simulink model "CNcs7"  (Simulink 6.2)
settings: Solver=ode4  SolverMode=SingleTasking  StartTime=0.0  StopTime=5  FixedStep=0.001  MaxStep=0.001  RelTol=1e-3  AbsTol=1e-3
undefined symbols (not defined in the file): alexlaw, bs_onoff, bs_scale, bsfsacrit, bsfsvcrit, cnsgain, fs_onoff, fs_scale, fsdelaycalc, ltdrk, phasicgain, pmcgain, pmctau2, pmctau3, saccrefract, saccsw, spgain, tonicgain, tvrD, tvrN, velnoise, velreconsw
libraries: simulink_extras x38, simulink x2
(part 5 of 5)

== system CNcs7/CN/LMLN  03/03/01/IM CN-LMLN/Saccade Enable/Enable Control/2 ms/leading edge detect ==
  note: leading edge detection
  in_1 : Inport  Port=1  LatchInput=off
  Abs : Abs  SaturateOnIntegerOverflow=on
  Derivative : Derivative
  Relational Operator : RelationalOperator  Operator===  InputSameDT=on
  Sign : Signum
  Threshold 1 : Constant
  out_1 : Outport
  wires:
  Abs/1 -> Derivative/1
  Derivative/1 -> Sign/1
  Sign/1 -> Relational Operator/1
  Threshold 1/1 -> Relational Operator/2
  Relational Operator/1 -> out_1/1
  in_1/1 -> Abs/1

== system CNcs7/CN/LMLN  03/03/01/IM CN-LMLN/Saccade Enable/Enable Control/2 ms/trailing edge detect ==
  note: trailing edge detection
  note: It is also possible to remove the SIGNUM function
      | and the '==', and replace them with a simple
      | switch with a threshold of (say) 150 or so.
  in_1 : Inport  Port=1  LatchInput=off
  Abs : Abs  SaturateOnIntegerOverflow=on
  Derivative : Derivative
  Relational Operator : RelationalOperator  Operator===  InputSameDT=on
  Sign : Signum
  Threshold 1 : Constant  Value=-1
  out_1 : Outport
  wires:
  in_1/1 -> Abs/1
  Relational Operator/1 -> out_1/1
  Threshold 1/1 -> Relational Operator/2
  Sign/1 -> Relational Operator/1
  Derivative/1 -> Sign/1
  Abs/1 -> Derivative/1

== system CNcs7/CN/LMLN  03/03/01/IM CN-LMLN/Saccade Enable/Enable Control/50 ms/SampHold?2 ==
  note: When "S/H?" is LOW, then "Input" is switched directly to the
      | output ("sample").  When "S/H?" is HIGH, the current output is
      | maintained ("hold").
  Input : Inport  Port=1  LatchInput=off
  S/H? : Inport  Port=2  LatchInput=off
  Memory : Memory  Orientation=left
  Sign : Signum
  Switch2 : Switch  Threshold=0.5  SaturateOnIntegerOverflow=on  InputSameDT=on
  output : Outport
  wires:
  S/H?/1 -> Sign/1
  Sign/1 -> Switch2/2
  Input/1 -> Switch2/3
  Switch2/1 -> Memory/1, output/1
  Memory/1 -> Switch2/1

== system CNcs7/CN/LMLN  03/03/01/IM CN-LMLN/Saccade Enable/Enable Control/50 ms/leading edge detect ==
  note: leading edge detection
  in_1 : Inport  Port=1  LatchInput=off
  Abs : Abs  SaturateOnIntegerOverflow=on
  Derivative : Derivative
  Relational Operator : RelationalOperator  Operator===  InputSameDT=on
  Sign : Signum
  Threshold 1 : Constant
  out_1 : Outport
  wires:
  in_1/1 -> Abs/1
  Relational Operator/1 -> out_1/1
  Threshold 1/1 -> Relational Operator/2
  Sign/1 -> Relational Operator/1
  Derivative/1 -> Sign/1
  Abs/1 -> Derivative/1

== system CNcs7/CN/LMLN  03/03/01/IM CN-LMLN/Saccade Enable/Enable Control/50 ms/trailing edge detect ==
  note: It is also possible to remove the SIGNUM function
      | and the '==', and replace them with a simple
      | switch with a threshold of (say) 150 or so.
  note: trailing edge detection
  in_1 : Inport  Port=1  LatchInput=off
  Abs : Abs  SaturateOnIntegerOverflow=on
  Derivative : Derivative
  Relational Operator : RelationalOperator  Operator===  InputSameDT=on
  Sign : Signum
  Threshold 1 : Constant  Value=-1
  out_1 : Outport
  wires:
  Abs/1 -> Derivative/1
  Derivative/1 -> Sign/1
  Sign/1 -> Relational Operator/1
  Threshold 1/1 -> Relational Operator/2
  Relational Operator/1 -> out_1/1
  in_1/1 -> Abs/1

== system CNcs7/CN/LMLN  03/03/01/IM CN-LMLN/Saccade Enable/Enable Control/ECPY Timing/leading edge detect ==
  note: It is also possible to remove the SIGNUM function
      | and the '==', and replace them with a simple
      | switch with a threshold of (say) 150 or so.
  note: leading edge detection
  in_1 : Inport  Port=1  LatchInput=off
  Abs : Abs  SaturateOnIntegerOverflow=on
  Derivative : Derivative
  Relational Operator : RelationalOperator  Operator===  InputSameDT=on
  Sign : Signum
  Threshold 1 : Constant
  out_1 : Outport
  wires:
  Abs/1 -> Derivative/1
  Derivative/1 -> Sign/1
  Sign/1 -> Relational Operator/1
  Threshold 1/1 -> Relational Operator/2
  Relational Operator/1 -> out_1/1
  in_1/1 -> Abs/1

== system CNcs7/CN/LMLN  03/03/01/IM CN-LMLN/Saccade Enable/Enable Control/ECPY Timing/leading edge detect1 ==
  note: leading edge detection
  note: It is also possible to remove the SIGNUM function
      | and the '==', and replace them with a simple
      | switch with a threshold of (say) 150 or so.
  in_1 : Inport  Port=1  LatchInput=off
  Abs : Abs  SaturateOnIntegerOverflow=on
  Derivative : Derivative
  Relational Operator : RelationalOperator  Operator===  InputSameDT=on
  Sign : Signum
  Threshold 1 : Constant
  out_1 : Outport
  wires:
  in_1/1 -> Abs/1
  Relational Operator/1 -> out_1/1
  Threshold 1/1 -> Relational Operator/2
  Sign/1 -> Relational Operator/1
  Derivative/1 -> Sign/1
  Abs/1 -> Derivative/1

== system CNcs7/CN/LMLN  03/03/01/IM CN-LMLN/Saccade Enable/Enable Control/ECPY Timing/trailing edge detect ==
  note: trailing edge detection
  note: It is also possible to remove the SIGNUM function
      | and the '==', and replace them with a simple
      | switch with a threshold of (say) 150 or so.
  in_1 : Inport  Port=1  LatchInput=off
  Abs : Abs  SaturateOnIntegerOverflow=on
  Derivative : Derivative
  Relational Operator : RelationalOperator  Operator===  InputSameDT=on
  Sign : Signum
  Threshold 1 : Constant  Value=-1
  out_1 : Outport
  wires:
  in_1/1 -> Abs/1
  Relational Operator/1 -> out_1/1
  Threshold 1/1 -> Relational Operator/2
  Sign/1 -> Relational Operator/1
  Derivative/1 -> Sign/1
  Abs/1 -> Derivative/1

== system CNcs7/CN/LMLN  03/03/01/IM CN-LMLN/Saccade Enable/Enable Control/event timer1/SampHold?1 ==
  note: When "S/H?" is LOW, then "Input" is switched directly to the
      | output ("sample").  When "S/H?" is HIGH, the current output is
      | maintained ("hold").
  Input : Inport  Port=1  LatchInput=off
  S/H? : Inport  Port=2  LatchInput=off
  Memory : Memory  Orientation=left
  Sign : Signum
  Switch2 : Switch  Threshold=0.5  SaturateOnIntegerOverflow=on  InputSameDT=on
  output : Outport
  wires:
  Input/1 -> Switch2/3
  Memory/1 -> Switch2/1
  S/H?/1 -> Sign/1
  Sign/1 -> Switch2/2
  Switch2/1 -> output/1, Memory/1

== system CNcs7/CN/LMLN  03/03/01/IM CN-LMLN/Saccade Enable/Enable Control/event timer1/leading edge detect ==
  note: leading edge detection
  note: It is also possible to remove the SIGNUM function
      | and the '==', and replace them with a simple
      | switch with a threshold of (say) 150 or so.
  in_1 : Inport  Port=1  LatchInput=off
  Abs : Abs  SaturateOnIntegerOverflow=on
  Derivative : Derivative
  Relational Operator : RelationalOperator  Operator===  InputSameDT=on
  Sign : Signum
  Threshold 1 : Constant
  out_1 : Outport
  wires:
  in_1/1 -> Abs/1
  Relational Operator/1 -> out_1/1
  Threshold 1/1 -> Relational Operator/2
  Sign/1 -> Relational Operator/1
  Derivative/1 -> Sign/1
  Abs/1 -> Derivative/1

== system CNcs7/CN/LMLN  03/03/01/IM CN-LMLN/Saccade Enable/Enable Control/event timer1/trailing edge detect ==
  note: It is also possible to remove the SIGNUM function
      | and the '==', and replace them with a simple
      | switch with a threshold of (say) 150 or so.
  note: trailing edge detection
  in_1 : Inport  Port=1  LatchInput=off
  Abs : Abs  SaturateOnIntegerOverflow=on
  Derivative : Derivative
  Relational Operator : RelationalOperator  Operator===  InputSameDT=on
  Sign : Signum
  Threshold 1 : Constant  Value=-1
  out_1 : Outport
  wires:
  Abs/1 -> Derivative/1
  Derivative/1 -> Sign/1
  Sign/1 -> Relational Operator/1
  Threshold 1/1 -> Relational Operator/2
  Relational Operator/1 -> out_1/1
  in_1/1 -> Abs/1

== system CNcs7/CN/LMLN  03/03/01/IM CN-LMLN/Saccade Enable/LN FPh Gen/event timer1/SampHold?1 ==
  note: When "S/H?" is LOW, then "Input" is switched directly to the
      | output ("sample").  When "S/H?" is HIGH, the current output is
      | maintained ("hold").
  Input : Inport  Port=1  LatchInput=off
  S/H? : Inport  Port=2  LatchInput=off
  Memory : Memory  Orientation=left
  Sign : Signum
  Switch2 : Switch  Threshold=0.5  SaturateOnIntegerOverflow=on  InputSameDT=on
  output : Outport
  wires:
  Input/1 -> Switch2/3
  Memory/1 -> Switch2/1
  S/H?/1 -> Sign/1
  Sign/1 -> Switch2/2
  Switch2/1 -> output/1, Memory/1

== system CNcs7/CN/LMLN  03/03/01/IM CN-LMLN/Saccade Enable/LN FPh Gen/event timer1/leading edge detect ==
  note: leading edge detection
  note: It is also possible to remove the SIGNUM function
      | and the '==', and replace them with a simple
      | switch with a threshold of (say) 150 or so.
  in_1 : Inport  Port=1  LatchInput=off
  Abs : Abs  SaturateOnIntegerOverflow=on
  Derivative : Derivative
  Relational Operator : RelationalOperator  Operator===  InputSameDT=on
  Sign : Signum
  Threshold 1 : Constant
  out_1 : Outport
  wires:
  in_1/1 -> Abs/1
  Relational Operator/1 -> out_1/1
  Threshold 1/1 -> Relational Operator/2
  Sign/1 -> Relational Operator/1
  Derivative/1 -> Sign/1
  Abs/1 -> Derivative/1

== system CNcs7/CN/LMLN  03/03/01/IM CN-LMLN/Saccade Enable/LN FPh Gen/event timer1/trailing edge detect ==
  note: It is also possible to remove the SIGNUM function
      | and the '==', and replace them with a simple
      | switch with a threshold of (say) 150 or so.
  note: trailing edge detection
  in_1 : Inport  Port=1  LatchInput=off
  Abs : Abs  SaturateOnIntegerOverflow=on
  Derivative : Derivative
  Relational Operator : RelationalOperator  Operator===  InputSameDT=on
  Sign : Signum
  Threshold 1 : Constant  Value=-1
  out_1 : Outport
  wires:
  Abs/1 -> Derivative/1
  Derivative/1 -> Sign/1
  Sign/1 -> Relational Operator/1
  Threshold 1/1 -> Relational Operator/2
  Relational Operator/1 -> out_1/1
  in_1/1 -> Abs/1

== system CNcs7/CN/LMLN  03/03/01/IM CN-LMLN/Saccade Enable/Ret FB sample/event timer2/SampHold?1 ==
  note: When "S/H?" is LOW, then "Input" is switched directly to the
      | output ("sample").  When "S/H?" is HIGH, the current output is
      | maintained ("hold").
  Input : Inport  Port=1  LatchInput=off
  S/H? : Inport  Port=2  LatchInput=off
  Memory : Memory  Orientation=left
  Sign : Signum
  Switch2 : Switch  Threshold=0.5  SaturateOnIntegerOverflow=on  InputSameDT=on
  output : Outport
  wires:
  Switch2/1 -> Memory/1, output/1
  Sign/1 -> Switch2/2
  S/H?/1 -> Sign/1
  Memory/1 -> Switch2/1
  Input/1 -> Switch2/3

== system CNcs7/CN/LMLN  03/03/01/IM CN-LMLN/Saccade Enable/Ret FB sample/event timer2/leading edge detect ==
  note: It is also possible to remove the SIGNUM function
      | and the '==', and replace them with a simple
      | switch with a threshold of (say) 150 or so.
  note: leading edge detection
  in_1 : Inport  Port=1  LatchInput=off
  Abs : Abs  SaturateOnIntegerOverflow=on
  Derivative : Derivative
  Relational Operator : RelationalOperator  Operator===  InputSameDT=on
  Sign : Signum
  Threshold 1 : Constant
  out_1 : Outport
  wires:
  Abs/1 -> Derivative/1
  Derivative/1 -> Sign/1
  Sign/1 -> Relational Operator/1
  Threshold 1/1 -> Relational Operator/2
  Relational Operator/1 -> out_1/1
  in_1/1 -> Abs/1

== system CNcs7/CN/LMLN  03/03/01/IM CN-LMLN/Saccade Enable/Ret FB sample/event timer2/trailing edge detect ==
  note: trailing edge detection
  note: It is also possible to remove the SIGNUM function
      | and the '==', and replace them with a simple
      | switch with a threshold of (say) 150 or so.
  in_1 : Inport  Port=1  LatchInput=off
  Abs : Abs  SaturateOnIntegerOverflow=on
  Derivative : Derivative
  Relational Operator : RelationalOperator  Operator===  InputSameDT=on
  Sign : Signum
  Threshold 1 : Constant  Value=-1
  out_1 : Outport
  wires:
  in_1/1 -> Abs/1
  Relational Operator/1 -> out_1/1
  Threshold 1/1 -> Relational Operator/2
  Sign/1 -> Relational Operator/1
  Derivative/1 -> Sign/1
  Abs/1 -> Derivative/1

== system CNcs7/CN/LMLN  03/03/01/IM CN-LMLN/Saccade Enable/Ret FB sample/event timer3/SampHold?1 ==
  note: When "S/H?" is LOW, then "Input" is switched directly to the
      | output ("sample").  When "S/H?" is HIGH, the current output is
      | maintained ("hold").
  Input : Inport  Port=1  LatchInput=off
  S/H? : Inport  Port=2  LatchInput=off
  Memory : Memory  Orientation=left
  Sign : Signum
  Switch2 : Switch  Threshold=0.5  SaturateOnIntegerOverflow=on  InputSameDT=on
  output : Outport
  wires:
  Input/1 -> Switch2/3
  Memory/1 -> Switch2/1
  S/H?/1 -> Sign/1
  Sign/1 -> Switch2/2
  Switch2/1 -> output/1, Memory/1

== system CNcs7/CN/LMLN  03/03/01/IM CN-LMLN/Saccade Enable/Ret FB sample/event timer3/leading edge detect ==
  note: leading edge detection
  note: It is also possible to remove the SIGNUM function
      | and the '==', and replace them with a simple
      | switch with a threshold of (say) 150 or so.
  in_1 : Inport  Port=1  LatchInput=off
  Abs : Abs  SaturateOnIntegerOverflow=on
  Derivative : Derivative
  Relational Operator : RelationalOperator  Operator===  InputSameDT=on
  Sign : Signum
  Threshold 1 : Constant
  out_1 : Outport
  wires:
  in_1/1 -> Abs/1
  Relational Operator/1 -> out_1/1
  Threshold 1/1 -> Relational Operator/2
  Sign/1 -> Relational Operator/1
  Derivative/1 -> Sign/1
  Abs/1 -> Derivative/1

== system CNcs7/CN/LMLN  03/03/01/IM CN-LMLN/Saccade Enable/Ret FB sample/event timer3/trailing edge detect ==
  note: It is also possible to remove the SIGNUM function
      | and the '==', and replace them with a simple
      | switch with a threshold of (say) 150 or so.
  note: trailing edge detection
  in_1 : Inport  Port=1  LatchInput=off
  Abs : Abs  SaturateOnIntegerOverflow=on
  Derivative : Derivative
  Relational Operator : RelationalOperator  Operator===  InputSameDT=on
  Sign : Signum
  Threshold 1 : Constant  Value=-1
  out_1 : Outport
  wires:
  Abs/1 -> Derivative/1
  Derivative/1 -> Sign/1
  Sign/1 -> Relational Operator/1
  Threshold 1/1 -> Relational Operator/2
  Relational Operator/1 -> out_1/1
  in_1/1 -> Abs/1

== system CNcs7/CN/LMLN  03/03/01/IM CN-LMLN/Saccade Motor Commmand/TCHNG Override/event timer2/SampHold?1 ==
  note: When "S/H?" is LOW, then "Input" is switched directly to the
      | output ("sample").  When "S/H?" is HIGH, the current output is
      | maintained ("hold").
  Input : Inport  Port=1  LatchInput=off
  S/H? : Inport  Port=2  LatchInput=off
  Memory : Memory  Orientation=left
  Sign : Signum
  Switch2 : Switch  Threshold=0.5  SaturateOnIntegerOverflow=on  InputSameDT=on
  output : Outport
  wires:
  Switch2/1 -> Memory/1, output/1
  Sign/1 -> Switch2/2
  S/H?/1 -> Sign/1
  Memory/1 -> Switch2/1
  Input/1 -> Switch2/3

== system CNcs7/CN/LMLN  03/03/01/IM CN-LMLN/Saccade Motor Commmand/TCHNG Override/event timer2/leading edge detect ==
  note: It is also possible to remove the SIGNUM function
      | and the '==', and replace them with a simple
      | switch with a threshold of (say) 150 or so.
  note: leading edge detection
  in_1 : Inport  Port=1  LatchInput=off
  Abs : Abs  SaturateOnIntegerOverflow=on
  Derivative : Derivative
  Relational Operator : RelationalOperator  Operator===  InputSameDT=on
  Sign : Signum
  Threshold 1 : Constant
  out_1 : Outport
  wires:
  Abs/1 -> Derivative/1
  Derivative/1 -> Sign/1
  Sign/1 -> Relational Operator/1
  Threshold 1/1 -> Relational Operator/2
  Relational Operator/1 -> out_1/1
  in_1/1 -> Abs/1

== system CNcs7/CN/LMLN  03/03/01/IM CN-LMLN/Saccade Motor Commmand/TCHNG Override/event timer2/trailing edge detect ==
  note: trailing edge detection
  note: It is also possible to remove the SIGNUM function
      | and the '==', and replace them with a simple
      | switch with a threshold of (say) 150 or so.
  in_1 : Inport  Port=1  LatchInput=off
  Abs : Abs  SaturateOnIntegerOverflow=on
  Derivative : Derivative
  Relational Operator : RelationalOperator  Operator===  InputSameDT=on
  Sign : Signum
  Threshold 1 : Constant  Value=-1
  out_1 : Outport
  wires:
  in_1/1 -> Abs/1
  Relational Operator/1 -> out_1/1
  Threshold 1/1 -> Relational Operator/2
  Sign/1 -> Relational Operator/1
  Derivative/1 -> Sign/1
  Abs/1 -> Derivative/1

== system CNcs7/CN/LMLN  03/03/01/IM CN-LMLN/BS/FS Logic/BS Enable1/BS Timing/event timer2/SampHold?1 ==
  note: When "S/H?" is LOW, then "Input" is switched directly to the
      | output ("sample").  When "S/H?" is HIGH, the current output is
      | maintained ("hold").
  Input : Inport  Port=1  LatchInput=off
  S/H? : Inport  Port=2  LatchInput=off
  Memory : Memory  Orientation=left
  Sign : Signum
  Switch2 : Switch  Threshold=0.5  SaturateOnIntegerOverflow=on  InputSameDT=on
  output : Outport
  wires:
  Switch2/1 -> Memory/1, output/1
  Sign/1 -> Switch2/2
  S/H?/1 -> Sign/1
  Memory/1 -> Switch2/1
  Input/1 -> Switch2/3

== system CNcs7/CN/LMLN  03/03/01/IM CN-LMLN/BS/FS Logic/BS Enable1/BS Timing/event timer2/leading edge detect ==
  note: It is also possible to remove the SIGNUM function
      | and the '==', and replace them with a simple
      | switch with a threshold of (say) 150 or so.
  note: leading edge detection
  in_1 : Inport  Port=1  LatchInput=off
  Abs : Abs  SaturateOnIntegerOverflow=on
  Derivative : Derivative
  Relational Operator : RelationalOperator  Operator===  InputSameDT=on
  Sign : Signum
  Threshold 1 : Constant
  out_1 : Outport
  wires:
  Abs/1 -> Derivative/1
  Derivative/1 -> Sign/1
  Sign/1 -> Relational Operator/1
  Threshold 1/1 -> Relational Operator/2
  Relational Operator/1 -> out_1/1
  in_1/1 -> Abs/1

== system CNcs7/CN/LMLN  03/03/01/IM CN-LMLN/BS/FS Logic/BS Enable1/BS Timing/event timer2/trailing edge detect ==
  note: trailing edge detection
  note: It is also possible to remove the SIGNUM function
      | and the '==', and replace them with a simple
      | switch with a threshold of (say) 150 or so.
  in_1 : Inport  Port=1  LatchInput=off
  Abs : Abs  SaturateOnIntegerOverflow=on
  Derivative : Derivative
  Relational Operator : RelationalOperator  Operator===  InputSameDT=on
  Sign : Signum
  Threshold 1 : Constant  Value=-1
  out_1 : Outport
  wires:
  in_1/1 -> Abs/1
  Relational Operator/1 -> out_1/1
  Threshold 1/1 -> Relational Operator/2
  Sign/1 -> Relational Operator/1
  Derivative/1 -> Sign/1
  Abs/1 -> Derivative/1

== system CNcs7/CN/LMLN  03/03/01/IM CN-LMLN/BS/FS Logic/FS Enable/FS Timing/event timer2/SampHold?1 ==
  note: When "S/H?" is LOW, then "Input" is switched directly to the
      | output ("sample").  When "S/H?" is HIGH, the current output is
      | maintained ("hold").
  Input : Inport  Port=1  LatchInput=off
  S/H? : Inport  Port=2  LatchInput=off
  Memory : Memory  Orientation=left
  Sign : Signum
  Switch2 : Switch  Threshold=0.5  SaturateOnIntegerOverflow=on  InputSameDT=on
  output : Outport
  wires:
  Input/1 -> Switch2/3
  Memory/1 -> Switch2/1
  S/H?/1 -> Sign/1
  Sign/1 -> Switch2/2
  Switch2/1 -> output/1, Memory/1

== system CNcs7/CN/LMLN  03/03/01/IM CN-LMLN/BS/FS Logic/FS Enable/FS Timing/event timer2/leading edge detect ==
  note: leading edge detection
  note: It is also possible to remove the SIGNUM function
      | and the '==', and replace them with a simple
      | switch with a threshold of (say) 150 or so.
  in_1 : Inport  Port=1  LatchInput=off
  Abs : Abs  SaturateOnIntegerOverflow=on
  Derivative : Derivative
  Relational Operator : RelationalOperator  Operator===  InputSameDT=on
  Sign : Signum
  Threshold 1 : Constant
  out_1 : Outport
  wires:
  in_1/1 -> Abs/1
  Relational Operator/1 -> out_1/1
  Threshold 1/1 -> Relational Operator/2
  Sign/1 -> Relational Operator/1
  Derivative/1 -> Sign/1
  Abs/1 -> Derivative/1

== system CNcs7/CN/LMLN  03/03/01/IM CN-LMLN/BS/FS Logic/FS Enable/FS Timing/event timer2/trailing edge detect ==
  note: It is also possible to remove the SIGNUM function
      | and the '==', and replace them with a simple
      | switch with a threshold of (say) 150 or so.
  note: trailing edge detection
  in_1 : Inport  Port=1  LatchInput=off
  Abs : Abs  SaturateOnIntegerOverflow=on
  Derivative : Derivative
  Relational Operator : RelationalOperator  Operator===  InputSameDT=on
  Sign : Signum
  Threshold 1 : Constant  Value=-1
  out_1 : Outport
  wires:
  Abs/1 -> Derivative/1
  Derivative/1 -> Sign/1
  Sign/1 -> Relational Operator/1
  Threshold 1/1 -> Relational Operator/2
  Relational Operator/1 -> out_1/1
  in_1/1 -> Abs/1
